simulink model "manualMPCRas"  (R2024a)
settings: Solver=FixedStepAuto  StartTime=0.0  StopTime=inf  FixedStep=Ts  RelTol=1e-3  EnableMultiTasking=on
values from neighbouring files (symbols this model uses):
  D = 0    [lqrandmpc.m]
  lamda = 0.1    [lqrandmpc.m]
  Nc = 1    [lqrandmpc.m]
  Np = 3    [lqrandmpc.m]
  Ts = 0.01    [load_example_QProblem.m]    (also in lqrandmpc.m)
undefined symbols (not defined in the file or in its folder): Phi_F, Phi_Phi, rad, s
libraries: raspberrypiBasiclib x8, simulink_extras x4, raspberrypiCommlib x3, aerolibconvert2 x2, eeGeneralControl x2, simulink x2
settings Model: ExtModeTrigDuration=2  Creator=Muham  LastModifiedBy=muham
settings SolverCC: PositivePriorityOrder=on  AutoInsertRateTranBlk=on
settings DataIOCC: SaveFormat=StructureWithTime  SaveOutput=off  SaveTime=off
settings OptimizationCC: ReuseModelBlockBuffer=off  EnhancedBackFolding=on  PassReuseOutputArgsAs=Individual arguments  ZeroExternalMemoryAtStartup=off  ZeroInternalMemoryAtStartup=off  MaxStackSize=64  OptimizeBlockOrder=speed  DifferentSizesBufferReuse=on  EfficientTunableParamExpr=on
settings DebuggingCC: ParameterTunabilityLossMsg=error  UnconnectedInputMsg=warning  UnconnectedOutputMsg=warning  UnconnectedLineMsg=warning
settings HardwareCC: ProdBitPerPointer=32  ProdBitPerSizeT=32  ProdBitPerPtrDiffT=32  ProdLargestAtomicInteger=Long  ProdLargestAtomicFloat=Double  ProdWordSize=32  ProdLongLongMode=on  ProdHWDeviceType=ARM Compatible->ARM Cortex
settings ModelReferenceCC: EnableRefExpFcnMdlSchedulingChecks=on
settings RTWCC: Description=Embedded Coder  SystemTargetFile=ert.tlc  HardwareBoard=Raspberry Pi  TLCOptions="-aInlineSetEventsForThisBaseRateFcn=TLC_FALSE -aSuppressMultiTaskScheduler=TLC_FALSE  -aRateBasedStepFcn=0"  TemplateMakefile=ert_default_tmf  Toolchain=GNU GCC Embedded Linux  BuildConfiguration=Faster Runs  GPUComputeCapability=3.5  DLArmComputeVersion=19.05
settings CodeAppCC: ForceParamTrailComments=on  IgnoreCustomStorageClasses=off  OperatorAnnotations=on  SimulinkDataObjDesc=on  SFDataObjDesc=on  InsertBlockDesc=on
settings ERTTargetCC: SupportContinuousTime=on  SupportVariableSizeSignals=on  ExtModeTransport=2  ExtModeStaticAlloc=on  ExtModeMexFile=ext_xcp  ExtModeIntrfLevel=Level2 - Open

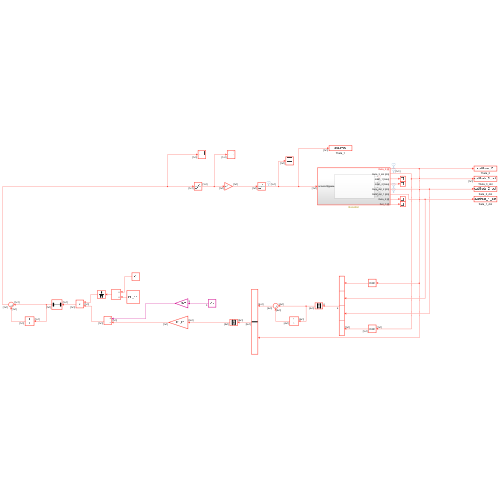
[thumbnail: Simulink's stored preview of the top-level diagram]
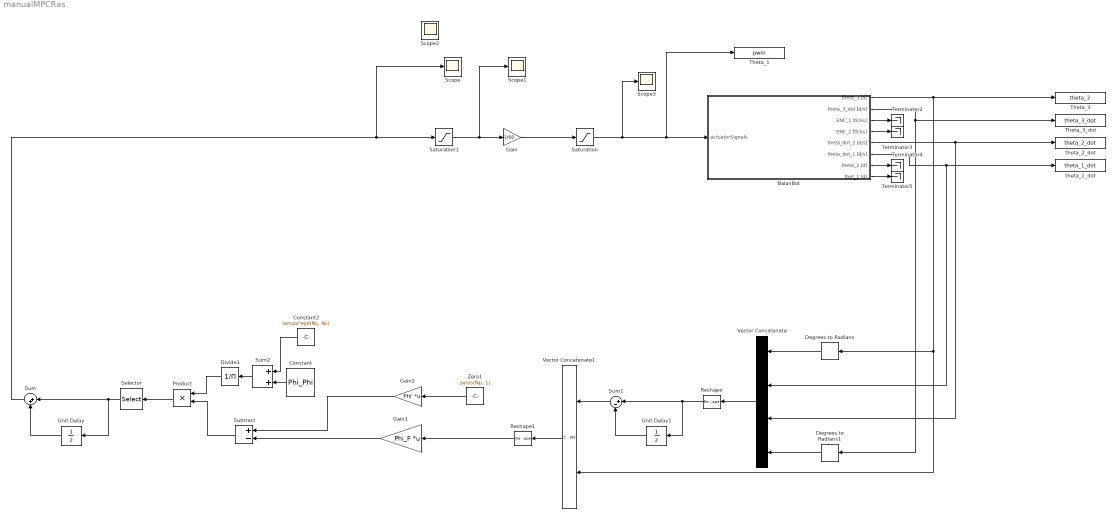
== system manualMPCRas ==
  BalanBot : Subsystem
  Constant : Constant  Value=Phi_Phi  SampleTime=-1
  Constant2 : Constant  Value=lamda*eye(Nc, Nc)  SampleTime=-1
  Degrees to Radians : simulink_extras/Transformations/Degrees to Radians
  Degrees to Radians1 : simulink_extras/Transformations/Degrees to Radians
  Divide1 : Product  Inputs=/
  Gain : Gain  Gain=1/60
  Gain1 : Gain  Gain=Phi_F  Multiplication=Matrix(K*u)
  Gain2 : Gain  Gain=Phi'  Multiplication=Matrix(K*u)
  Product : Product
  Reshape : Reshape  OutputDimensionality=Column vector (2-D)  OutputDimensions=[5,1]
  Reshape1 : Reshape  OutputDimensionality=Column vector (2-D)  OutputDimensions=[5,1]
  Saturation : Saturate  UpperLimit=1  LowerLimit=-1
  Saturation1 : Saturate  UpperLimit=200  LowerLimit=-200
  Scope{,1..3} (4 alike) : Scope
  Selector : Selector  InputPortWidth=Nc  IndexOptions=Index vector (dialog)  Indices=1  OutputSizes=1
  Subtract : Sum  Inputs=+-
  Sum : Sum  Inputs=|++
  Sum1 : Sum  Inputs=|+-
  Sum2 : Sum
  Terminator{2..5} (4 alike) : Terminator
  Theta_1 : ToWorkspace  VariableName=pwm  SaveFormat=Timeseries  SampleTime=Ts
  Theta_3 : ToWorkspace  VariableName=theta_3  SaveFormat=Timeseries  SampleTime=Ts
  Theta_3_dot : ToWorkspace  VariableName=theta_3_dot  SaveFormat=Timeseries  SampleTime=Ts
  Unit Delay : UnitDelay  SampleTime=-1  HasFrameUpgradeWarning=on
  Unit Delay1 : UnitDelay  SampleTime=-1  HasFrameUpgradeWarning=on
  Vector Concatenate : Concatenate  NumInputs=4
  Vector Concatenate1 : Concatenate
  Zero1 : Constant  Value=zeros(Np, 1)  OutDataTypeStr=Inherit: Inherit via back propagation
  theta_1_dot : ToWorkspace  VariableName=theta_1_dot  SaveFormat=Timeseries  SampleTime=Ts
  theta_2_dot : ToWorkspace  VariableName=theta_2_dot  SaveFormat=Timeseries  SampleTime=Ts
  wires:
  BalanBot/2(theta_3_dot [d/s]) -> Theta_3_dot/1, Degrees to Radians1/1
  Gain/1 -> Saturation/1
  Saturation1/1 -> Scope1/1, Gain/1
  BalanBot/3(ENC_1 [ticks]) -> Terminator2/1
  BalanBot/4(ENC_2 [ticks]) -> Terminator3/1
  BalanBot/5(theta_dot_2 [d/s]) -> Vector Concatenate/3, theta_2_dot/1
  BalanBot/6(theta_dot_1 [d/s]) -> Vector Concatenate/2, theta_1_dot/1
  BalanBot/7(theta_2 [d]) -> Terminator4/1
  BalanBot/8(thet_1 [d]) -> Terminator5/1
  BalanBot/1(theta_3 [d]) -> Vector Concatenate1/2, Degrees to Radians/1, Theta_3/1
  Selector/1 -> Unit Delay/1, Sum/1
  Unit Delay/1 -> Sum/2
  Reshape1/1 -> Gain1/1
  Unit Delay1/1 -> Sum1/2
  Reshape/1 -> Unit Delay1/1, Sum1/1
  Vector Concatenate/1 -> Reshape/1
  Sum1/1 -> Vector Concatenate1/1
  Vector Concatenate1/1 -> Reshape1/1
  Gain1/1 -> Subtract/2
  Gain2/1 -> Subtract/1
  Divide1/1 -> Product/1
  Subtract/1 -> Product/2
  Product/1 -> Selector/1
  Sum/1 -> Scope/1, Saturation1/1
  Degrees to Radians1/1 -> Vector Concatenate/4
  Degrees to Radians/1 -> Vector Concatenate/1
  Constant2/1 -> Sum2/1
  Constant/1 -> Sum2/2
  Sum2/1 -> Divide1/1
  Zero1/1 -> Gain2/1
  Saturation/1 -> Scope3/1, Theta_1/1, BalanBot/1(actuatorSignals)

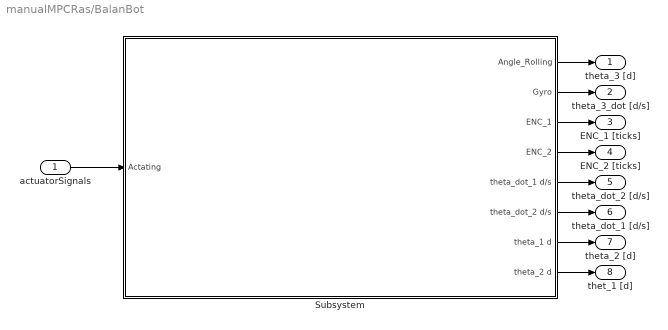
== system manualMPCRas/BalanBot ==
  actuatorSignals : Inport
  Subsystem : Subsystem  VariantControl=plantModel==2
  theta_3 [d] : Outport
  theta_3_dot [d/s] : Outport  Port=2
  ENC_1 [ticks] : Outport  Port=3
  ENC_2 [ticks] : Outport  Port=4
  theta_dot_2 [d/s] : Outport  Port=5
  theta_dot_1 [d/s] : Outport  Port=6
  theta_2 [d] : Outport  Port=7
  thet_1 [d] : Outport  Port=8
  wires:
  actuatorSignals/1 -> Subsystem/1(Actating)
  Subsystem/1(Angle_Rolling) -> theta_3 [d]/1
  Subsystem/2(Gyro) -> theta_3_dot [d/s]/1
  Subsystem/3(ENC_1) -> ENC_1 [ticks]/1
  Subsystem/4(ENC_2) -> ENC_2 [ticks]/1
  Subsystem/5(theta_dot_1 d/s) -> theta_dot_2 [d/s]/1
  Subsystem/6(theta_dot_2 d/s) -> theta_dot_1 [d/s]/1
  Subsystem/7(theta_1 d) -> theta_2 [d]/1
  Subsystem/8(theta_2 d) -> thet_1 [d]/1

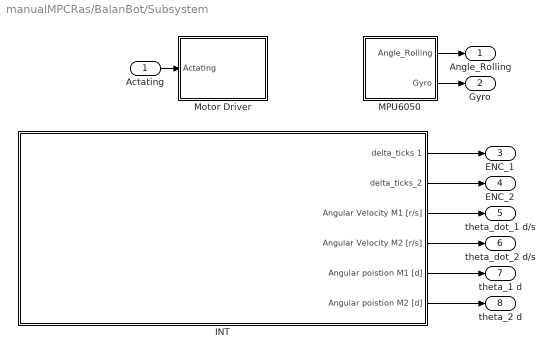
== system manualMPCRas/BalanBot/Subsystem ==
  Actating : Inport
  INT : Subsystem
  MPU6050 : Subsystem
  Motor Driver : Subsystem
  Angle_Rolling : Outport
  Gyro : Outport  Port=2
  ENC_1 : Outport  Port=3
  ENC_2 : Outport  Port=4
  theta_dot_1 d/s : Outport  Port=5
  theta_dot_2 d/s : Outport  Port=6
  theta_1 d : Outport  Port=7
  theta_2 d : Outport  Port=8
  wires:
  Actating/1 -> Motor Driver/1(Actating)
  INT/1(delta_ticks 1) -> ENC_1/1
  INT/2(delta_ticks_2) -> ENC_2/1
  INT/3(Angular Velocity M1 [r/s]) -> theta_dot_1 d/s/1
  INT/4(Angular Velocity M2 [r/s]) -> theta_dot_2 d/s/1
  INT/5(Angular poistion M1 [d]) -> theta_1 d/1
  INT/6(Angular poistion M2 [d]) -> theta_2 d/1
  MPU6050/2(Gyro) -> Gyro/1
  MPU6050/1(Angle_Rolling) -> Angle_Rolling/1

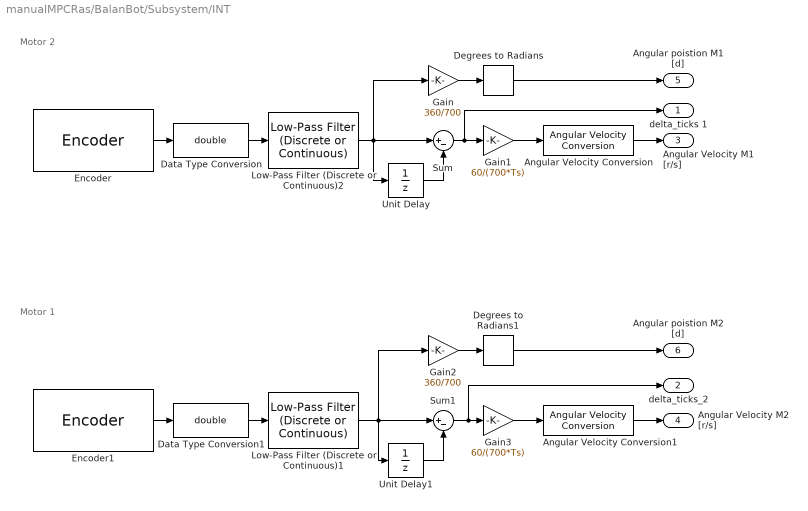
== system manualMPCRas/BalanBot/Subsystem/INT ==
  note: Motor 2
  note: Motor 1
  Angular Velocity Conversion : aerolibconvert2/Angular Velocity Conversion  IU=rpm  OU=rad/s
  Angular Velocity Conversion1 : aerolibconvert2/Angular Velocity Conversion  IU=rpm  OU=rad/s
  Data Type Conversion : DataTypeConversion  OutDataTypeStr=double  SaturateOnIntegerOverflow=off  RndMeth=Floor
  Data Type Conversion1 : DataTypeConversion  OutDataTypeStr=double  SaturateOnIntegerOverflow=off  RndMeth=Floor
  Degrees to Radians : simulink_extras/Transformations/Degrees to Radians
  Degrees to Radians1 : simulink_extras/Transformations/Degrees to Radians
  Encoder : raspberrypiBasiclib/Encoder  BoardProperty=Pi 4 Model B  InputA=GPIO 20  InputB=GPIO 21  Mode=No reset  SampleTime=-1
  Encoder1 : raspberrypiBasiclib/Encoder  BoardProperty=Pi 4 Model B  InputA=GPIO 26  InputB=GPIO 19  Mode=No reset  SampleTime=-1
  Gain : Gain  Gain=360/700
  Gain1 : Gain  Gain=60/(700*Ts)
  Gain2 : Gain  Gain=360/700
  Gain3 : Gain  Gain=60/(700*Ts)
  Low-Pass Filter (Discrete or Continuous)1 : eeGeneralControl/Low-Pass Filter (Discrete or Continuous)  K=1  T=Ts * 10  B=inf  A=-inf  init_option=Inherited from block input  x0=0  Ts=-1
  Low-Pass Filter (Discrete or Continuous)2 : eeGeneralControl/Low-Pass Filter (Discrete or Continuous)  K=1  T=Ts * 10  B=inf  A=-inf  init_option=Inherited from block input  x0=0  Ts=-1
  Sum : Sum  Inputs=|+-
  Sum1 : Sum  Inputs=|+-
  Unit Delay : UnitDelay  SampleTime=-1  HasFrameUpgradeWarning=on
  Unit Delay1 : UnitDelay  SampleTime=-1  HasFrameUpgradeWarning=on
  delta_ticks 1 : Outport
  delta_ticks_2 : Outport  Port=2
  Angular Velocity M1 [r/s] : Outport  Port=3
  Angular Velocity M2 [r/s] : Outport  Port=4
  Angular poistion M1 [d] : Outport  Port=5
  Angular poistion M2 [d] : Outport  Port=6
  wires:
  Encoder/1 -> Data Type Conversion/1
  Encoder1/1 -> Data Type Conversion1/1
  Data Type Conversion/1 -> Low-Pass Filter (Discrete or Continuous)2/1
  Sum/1 -> delta_ticks 1/1, Gain1/1
  Sum1/1 -> delta_ticks_2/1, Gain3/1
  Data Type Conversion1/1 -> Low-Pass Filter (Discrete or Continuous)1/1
  Low-Pass Filter (Discrete or Continuous)2/1 -> Gain/1, Sum/1, Unit Delay/1
  Unit Delay/1 -> Sum/2
  Gain1/1 -> Angular Velocity Conversion/1
  Angular Velocity Conversion/1 -> Angular Velocity M1 [r/s]/1
  Gain/1 -> Degrees to Radians/1
  Degrees to Radians/1 -> Angular poistion M1 [d]/1
  Angular Velocity Conversion1/1 -> Angular Velocity M2 [r/s]/1
  Gain3/1 -> Angular Velocity Conversion1/1
  Gain2/1 -> Degrees to Radians1/1
  Unit Delay1/1 -> Sum1/2
  Low-Pass Filter (Discrete or Continuous)1/1 -> Gain2/1, Sum1/1, Unit Delay1/1
  Degrees to Radians1/1 -> Angular poistion M2 [d]/1

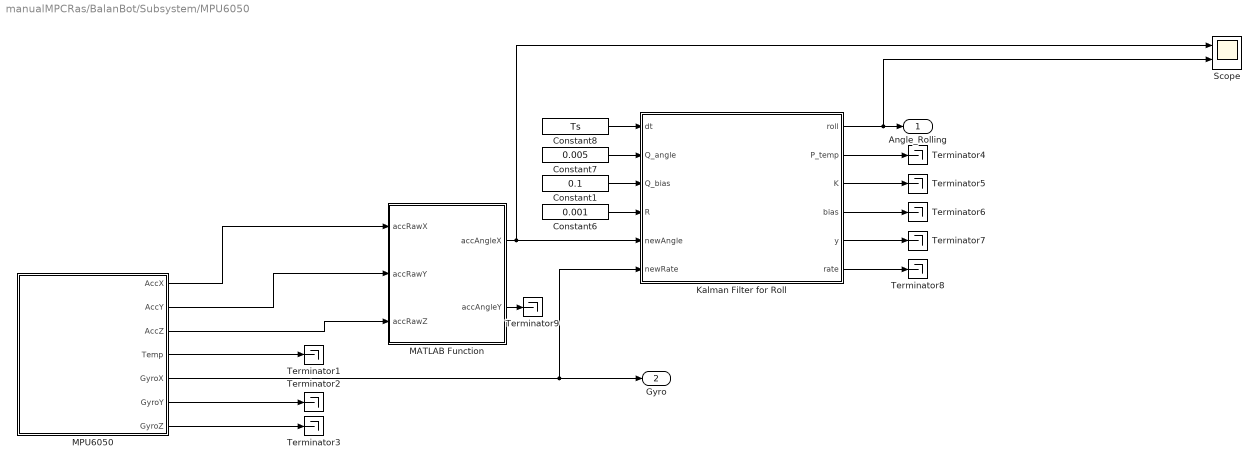
== system manualMPCRas/BalanBot/Subsystem/MPU6050 ==
  Constant1 : Constant  Value=0.1
  Constant6 : Constant  Value=0.001
  Constant7 : Constant  Value=0.005
  Constant8 : Constant  Value=Ts
  Kalman Filter for Roll : MATLAB Function  TreatAsAtomicUnit=on
  MATLAB Function : MATLAB Function  TreatAsAtomicUnit=on
  MPU6050 : Subsystem  TreatAsAtomicUnit=on
  Scope : Scope  NumInputPorts=2
  Terminator{1..9} (9 alike) : Terminator
  Angle_Rolling : Outport
  Gyro : Outport  Port=2
  wires:
  MPU6050/7(GyroZ) -> Terminator3/1
  MPU6050/5(GyroX) -> Kalman Filter for Roll/6(newRate), Gyro/1
  MPU6050/2(AccY) -> MATLAB Function/2(accRawY)
  MPU6050/3(AccZ) -> MATLAB Function/3(accRawZ)
  MPU6050/4(Temp) -> Terminator1/1
  MPU6050/1(AccX) -> MATLAB Function/1(accRawX)
  Constant8/1 -> Kalman Filter for Roll/1(dt)
  Constant7/1 -> Kalman Filter for Roll/2(Q_angle)
  Constant1/1 -> Kalman Filter for Roll/3(Q_bias)
  Constant6/1 -> Kalman Filter for Roll/4(R)
  Kalman Filter for Roll/1(roll) -> Scope/2, Angle_Rolling/1
  Kalman Filter for Roll/2(P_temp) -> Terminator4/1
  Kalman Filter for Roll/3(K) -> Terminator5/1
  Kalman Filter for Roll/4(bias) -> Terminator6/1
  Kalman Filter for Roll/5(y) -> Terminator7/1
  Kalman Filter for Roll/6(rate) -> Terminator8/1
  MATLAB Function/1(accAngleX) -> Scope/1, Kalman Filter for Roll/5(newAngle)
  MPU6050/6(GyroY) -> Terminator2/1
  MATLAB Function/2(accAngleY) -> Terminator9/1

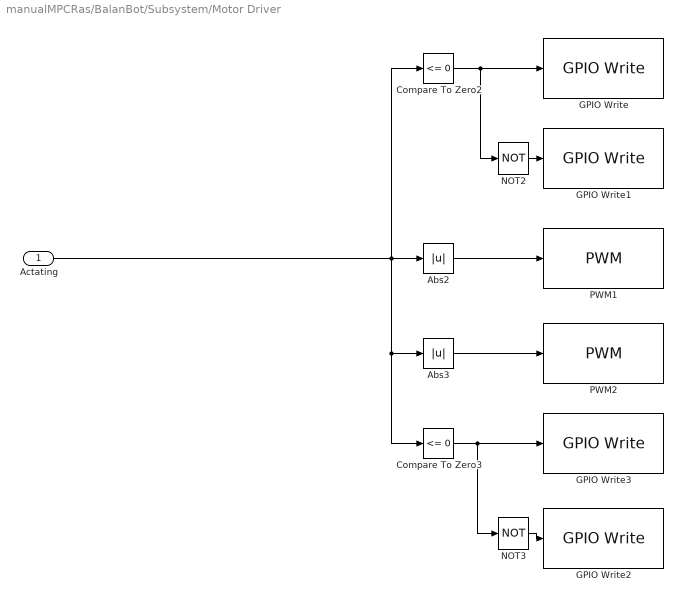
== system manualMPCRas/BalanBot/Subsystem/Motor Driver ==
  Actating : Inport
  Abs2 : Abs  SaturateOnIntegerOverflow=off
  Abs3 : Abs  SaturateOnIntegerOverflow=off
  Compare To Zero2 : simulink/Logic and Bit Operations/Compare To Zero  relop=<=  OutDataTypeStr=boolean
  Compare To Zero3 : simulink/Logic and Bit Operations/Compare To Zero  relop=<=  OutDataTypeStr=boolean
  GPIO Write : raspberrypiBasiclib/GPIO Write  board=Pi 4 Model B  gpio=27  direction=Output  blockPlatform=Raspberry Pi
  GPIO Write1 : raspberrypiBasiclib/GPIO Write  board=Pi 4 Model B  gpio=22  direction=Output  blockPlatform=Raspberry Pi
  GPIO Write2 : raspberrypiBasiclib/GPIO Write  board=Pi 4 Model B  gpio=15  direction=Output  blockPlatform=Raspberry Pi
  GPIO Write3 : raspberrypiBasiclib/GPIO Write  board=Pi 4 Model B  gpio=18  direction=Output  blockPlatform=Raspberry Pi
  NOT2 : Logic  Operator=NOT  IconShape=distinctive  AllPortsSameDT=off  OutDataTypeStr=boolean
  NOT3 : Logic  Operator=NOT  IconShape=distinctive  AllPortsSameDT=off  OutDataTypeStr=boolean
  PWM1 : raspberrypiBasiclib/PWM  board=Pi 4 Model B  Pin_=17  Frequency=1000  blockPlatform=Raspberry Pi
  PWM2 : raspberrypiBasiclib/PWM  board=Pi 4 Model B  Pin_=14  Frequency=1000  blockPlatform=Raspberry Pi
  wires:
  Compare To Zero2/1 -> GPIO Write/1, NOT2/1
  Abs3/1 -> PWM2/1
  NOT3/1 -> GPIO Write2/1
  Compare To Zero3/1 -> GPIO Write3/1, NOT3/1
  NOT2/1 -> GPIO Write1/1
  Abs2/1 -> PWM1/1
  Actating/1 -> Compare To Zero2/1, Abs2/1, Compare To Zero3/1, Abs3/1

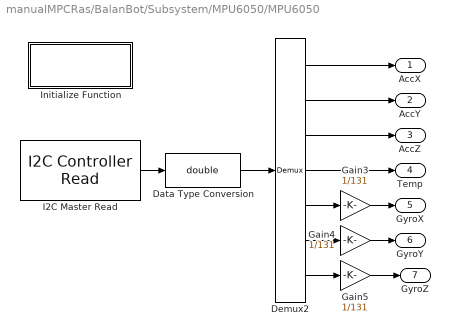
== system manualMPCRas/BalanBot/Subsystem/MPU6050/MPU6050 ==
  Data Type Conversion : DataTypeConversion  OutDataTypeStr=double  SaturateOnIntegerOverflow=off  RndMeth=Floor
  Demux2 : Demux  Outputs=7
  Gain3 : Gain  Gain=1/131
  Gain4 : Gain  Gain=1/131
  Gain5 : Gain  Gain=1/131
  I2C Master Read : raspberrypiCommlib/I2C Controller Read  BoardProperty=Pi 4 Model B  I2CModule=1  Mode=Master  SlaveAddress=hex2dec('68')  SlaveByteOrder=BigEndian  Direction=Receiver  RegisterAddressMode=on  RegisterAddress=hex2dec('3B')  SlaveDataType=int16  DataLength=7  NoAck=off  RepeatedStart=off  OutputStatus=off  SampleTime=-1
  Initialize Function : Subsystem  TreatAsAtomicUnit=on
  AccX : Outport
  AccY : Outport  Port=2
  AccZ : Outport  Port=3
  Temp : Outport  Port=4
  GyroX : Outport  Port=5
  GyroY : Outport  Port=6
  GyroZ : Outport  Port=7
  wires:
  Data Type Conversion/1 -> Demux2/1
  Demux2/5 -> Gain3/1
  I2C Master Read/1 -> Data Type Conversion/1
  Demux2/4 -> Temp/1
  Demux2/6 -> Gain4/1
  Demux2/7 -> Gain5/1
  Demux2/1 -> AccX/1
  Demux2/2 -> AccY/1
  Demux2/3 -> AccZ/1
  Gain3/1 -> GyroX/1
  Gain4/1 -> GyroY/1
  Gain5/1 -> GyroZ/1

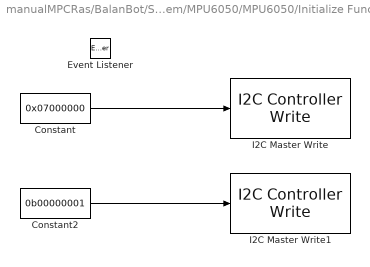
== system manualMPCRas/BalanBot/Subsystem/MPU6050/MPU6050/Initialize Function ==
  Constant : Constant  Value=0x07000000  SampleTime=-1
  Constant2 : Constant  Value=0b00000001  SampleTime=-1
  Event Listener : EventListener  DisableCoverage=on  EventName=reset
  I2C Master Write : raspberrypiCommlib/I2C Controller Write  BoardProperty=Pi 4 Model B  I2CModule=1  Mode=Master  SlaveAddress=uint8(hex2dec('68'))  SlaveByteOrder=BigEndian  Direction=Transmitter  RegisterAddressMode=on  RegisterAddress=uint8(hex2dec('19'))  SlaveDataType=uint8  DataLength=1  NoAck=off  RepeatedStart=off  OutputStatus=off
  I2C Master Write1 : raspberrypiCommlib/I2C Controller Write  BoardProperty=Pi 4 Model B  I2CModule=1  Mode=Master  SlaveAddress=hex2dec('68')  SlaveByteOrder=BigEndian  Direction=Transmitter  RegisterAddressMode=on  RegisterAddress=hex2dec('6B')  SlaveDataType=uint8  DataLength=1  NoAck=off  RepeatedStart=off  OutputStatus=off
  wires:
  Constant2/1 -> I2C Master Write1/1
  Constant/1 -> I2C Master Write/1

== matlab function manualMPCRas/BalanBot/Subsystem/MPU6050/MATLAB Function ==
  data: accRawX input; accAngleX output; accAngleY output; accRawY input; accRawZ input
function [accAngleX, accAngleY] = fcn(accRawX, accRawY, accRawZ)

%Converting the raw accel data from g values to accel about X and Y axis

accAngleX = atand(accRawY/sqrt(power(accRawX,2) + power(accRawZ,2)));
accAngleY = atand(-1*(accRawX/sqrt(power(accRawY,2) + power(accRawZ,2))));

end

== matlab function manualMPCRas/BalanBot/Subsystem/MPU6050/Kalman Filter for Roll ==
  data: dt input; roll output; Q_angle input; Q_bias input; R input; newAngle input; newRate input; P_temp output; K output; bias output; y output; rate output
function [roll, P_temp, K, bias, y, rate]  = kalFilterRoll(dt, Q_angle, Q_bias, R, newAngle, newRate)

persistent angle;
persistent P;


%Process Noise Convariance Matrix
Q = [Q_angle 0; 0 Q_bias] * dt;
F = [1  -dt; 0 1];
H = [1 0];
bias = 0.0;

rate = newRate - bias;

if isempty(angle)
    angle = 0;
else
    angle = angle + (dt * rate);
end 

roll = angle;

if isempty(P)
    P = [0, 0; 0, 0];
else
    P = F*P*F' + Q;
end 
P_temp = P;

S = H*P*H' + R;
K = (P_temp * H')/S;
y = newAngle - roll; 
roll = roll + K(1) * y;
bias = roll + K(2) * y;
angle = roll;

I = [1 0; 0 1];
P_temp = (I - K*H)*P_temp;
P = P_temp;

return 


end
